simulink model "Week3_Problem2"  (R2020b)
settings: Solver=FixedStepDiscrete  StartTime=0.0  StopTime=150  FixedStep=.1  RelTol=1e-3
undefined symbols (not defined in the file): DiscIntNeverNeededParam
libraries: simulink x1
settings Model: Creator=hp  LastModifiedBy=hp
settings DataIOCC: SaveFormat=Array  ReturnWorkspaceOutputs=off

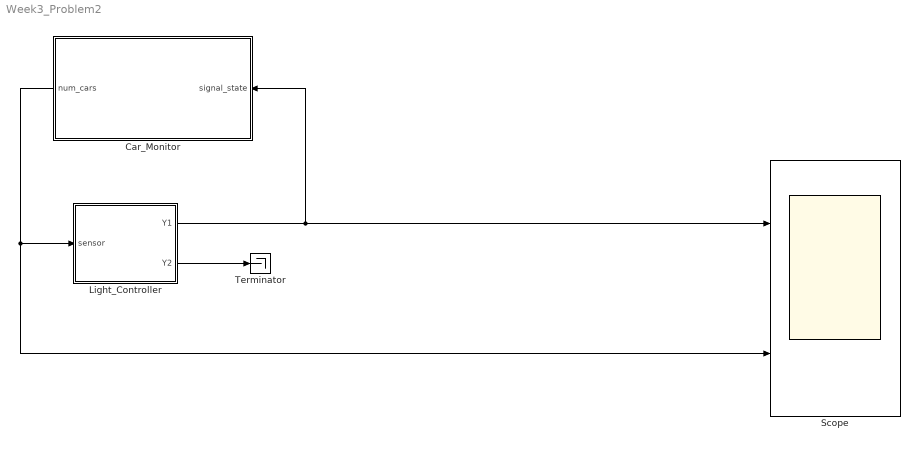
== system Week3_Problem2 ==
  Car_Monitor : Subsystem
  Light_Controller : Stateflow chart  TreatAsAtomicUnit=on
  Scope : Scope  NumInputPorts=2
  Terminator : Terminator
  wires:
  Light_Controller/1(Y1) -> Car_Monitor/1(signal_state), Scope/1
  Car_Monitor/1(num_cars) -> Scope/2, Light_Controller/1(sensor)
  Light_Controller/2(Y2) -> Terminator/1

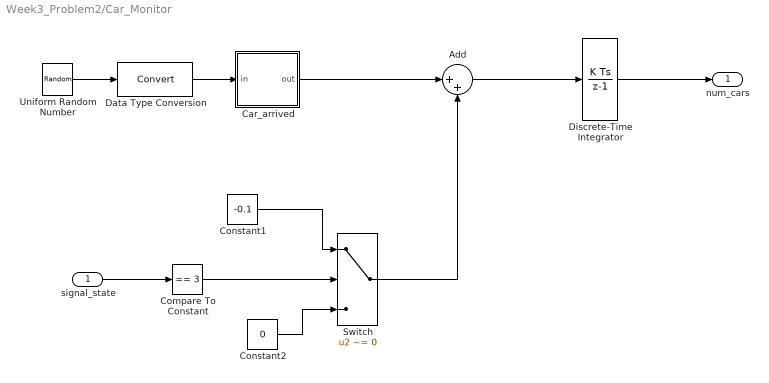
== system Week3_Problem2/Car_Monitor ==
  signal_state : Inport
  Add : Sum  Inputs=|++
  Car_arrived : Stateflow chart  TreatAsAtomicUnit=on
  Compare To Constant : simulink/Logic and Bit Operations/Compare To Constant  relop===  const=3  OutDataTypeStr=boolean  ZeroCross=off
  Constant1 : Constant  Value=-0.1
  Constant2 : Constant  Value=0
  Data Type Conversion : DataTypeConversion
  Discrete-Time Integrator : DiscreteIntegrator  SampleTime=-1  LimitOutput=on  LowerSaturationLimit=0  ICPrevOutput=DiscIntNeverNeededParam  ICPrevScaledInput=DiscIntNeverNeededParam
  Switch : Switch  Criteria=u2 ~= 0
  Uniform Random Number : UniformRandomNumber  Minimum=0  Maximum=100  Seed=177836  SampleTime=0
  num_cars : Outport  VectorParamsAs1DForOutWhenUnconnected=off
  wires:
  Constant1/1 -> Switch/1
  Constant2/1 -> Switch/3
  Discrete-Time Integrator/1 -> num_cars/1
  signal_state/1 -> Compare To Constant/1
  Compare To Constant/1 -> Switch/2
  Switch/1 -> Add/2
  Add/1 -> Discrete-Time Integrator/1
  Car_arrived/1(out) -> Add/1
  Data Type Conversion/1 -> Car_arrived/1(in)
  Uniform Random Number/1 -> Data Type Conversion/1

== stateflow chart Week3_Problem2/Light_Controller ==
  settings: stateMachineType=MOORE_MACHINE  executeAtInitialization=1  initializeOutput=1
  state Stop
    Y1 = red;
    Y2 = green;
  state StopForTraffic
    Y1 = red;
    Y2 = green;
  state GoToStop
    Y1 = yellow;
    Y2 = red;
  state StopToGo
    Y1 = red;
    Y2 = yellow;
  state Go
    Y1 = green;
    Y2 = red;
  (default) -> Stop
  GoToStop -> Stop : after (3,tick)
  Stop -> StopForTraffic : after(20,tick)
  StopForTraffic -> StopToGo : [sensor]
  Go -> GoToStop : after(10,tick)
  StopToGo -> Go : after(3,tick)
  data: green constant double =3; yellow constant double =2; red constant double =1; Y1 output double; Y2 output double; sensor input double

== stateflow chart Week3_Problem2/Car_Monitor/Car_arrived ==
  (default) -> (junction 2) : {out = in > 98;}
  data: in input int8; out output double
